simulink model "Torque_vectoring"  (R2023b)
settings: Solver=ode4  StartTime=0.0  StopTime=20  FixedStep=1e-3  RelTol=1e-3  EnableMultiTasking=on
undefined symbols (not defined in the file): A_vx, B_vx, D1, D2, LQR_DC, LQR_K, LQR_Vx_ref, N, P1, P2, par, V_ref
libraries: simulink x2, slpidlib x1
settings Model: Creator=bshyrokau  LastModifiedBy=india
settings SolverCC: AlgebraicLoopSolver=TrustRegion
settings DataIOCC: SaveOutput=off  SignalLogging=off  DSMLogging=off  SaveTime=off  ReturnWorkspaceOutputs=off
settings OptimizationCC: ReuseModelBlockBuffer=off  LifeSpan=inf
settings DebuggingCC: UnconnectedInputMsg=warning  UnconnectedOutputMsg=warning  UnconnectedLineMsg=warning  AllowSymbolicDim=off  SFUnexpectedBacktrackingDiag=warning  SFNoUnconditionalDefaultTransitionDiag=warning  SFExecutionAtInitializationDiag=none  ArithmeticOperatorsInVariantConditions=warning
settings ModelReferenceCC: EnableRefExpFcnMdlSchedulingChecks=on  PropagateSignalLabelsOutOfModel=off
settings SFSimCC: SimUseLocalCustomCode=off  CustomCodeUndefinedFunction=UseInterfaceOnly
settings RTWCC: RTWUseLocalCustomCode=off  DLArmComputeVersion=19.05
settings CodeAppCC: StateflowObjectComments=on
settings GRTTargetCC: TargetLangStandard=C89/C90 (ANSI)
settings ConfigComp: CovMetricSettings=dw  CovSaveCumulativeToWorkspaceVar=on  CovSaveSingleToWorkspaceVar=on  CovExternalEMLEnable=off
settings SimscapeCC: SimscapeNormalizeSystem=off
settings ConfigurationSet: Description=SimMechanics 2G

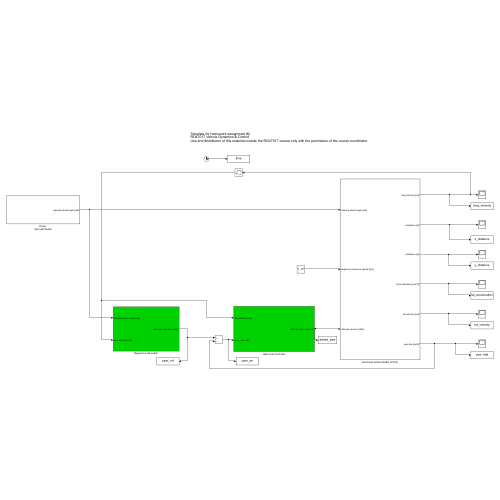
[thumbnail: Simulink's stored preview of the top-level diagram]
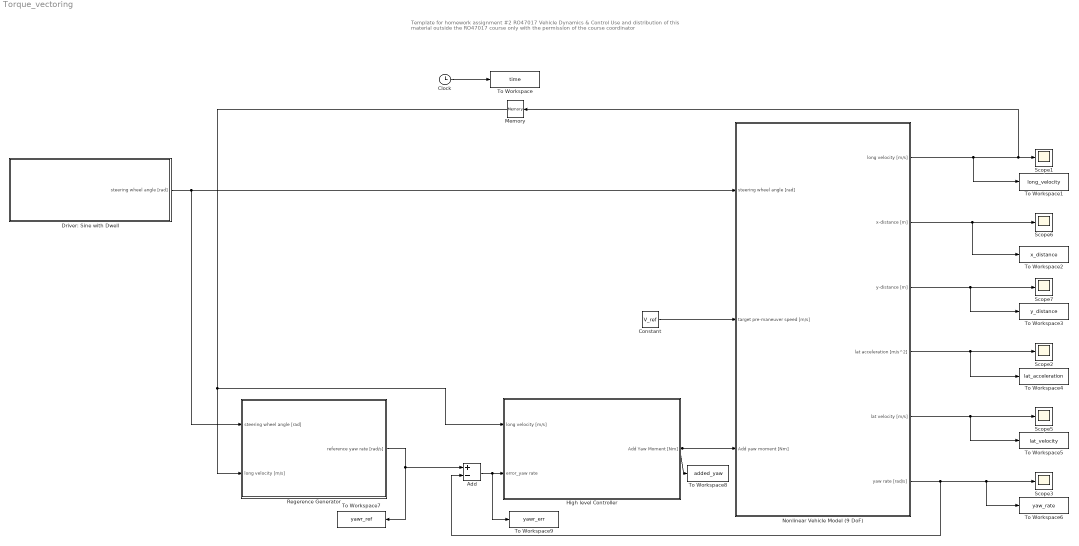
== system Torque_vectoring ==
  note: Template for homework assignment #2
      | RO47017 Vehicle Dynamics & Control
      | Use and distribution of this material outside the RO47017 course only with the permission of the course coordinator
  Add : Sum  Inputs=+-
  Clock : Clock
  Constant : Constant  Value=V_ref
  Driver: Sine with Dwell : Subsystem
  High level Controller : Subsystem
  Memory : Memory
  Nonlinear Vehicle Model (9 DoF) : Subsystem
      mask help: Simulink:masks:GenSFuncDesc_MD
      mask Help: eval('feval(''rtwprivate'',''rtwhelpview'',''rtw_sfcn_block'')');
  Regerence Generator : Subsystem
  Scope{1..3,5..7} (6 alike) : Scope
  To Workspace : ToWorkspace  VariableName=time  SampleTime=-1
  To Workspace1 : ToWorkspace  VariableName=long_velocity  SampleTime=-1
  To Workspace2 : ToWorkspace  VariableName=x_distance  SampleTime=-1
  To Workspace3 : ToWorkspace  VariableName=y_distance  SampleTime=-1
  To Workspace4 : ToWorkspace  VariableName=lat_acceleration  SampleTime=-1
  To Workspace5 : ToWorkspace  VariableName=lat_velocity  SampleTime=-1
  To Workspace6 : ToWorkspace  VariableName=yaw_rate  SampleTime=-1
  To Workspace7 : ToWorkspace  VariableName=yawr_ref  SampleTime=-1
  To Workspace8 : ToWorkspace  VariableName=added_yaw  SampleTime=-1
  To Workspace9 : ToWorkspace  VariableName=yawr_err  SampleTime=-1
  wires:
  Driver: Sine with Dwell/1(steering wheel angle [rad]) -> Regerence Generator/1(steering wheel angle [rad]), Nonlinear Vehicle Model (9 DoF)/1(steering wheel angle [rad])
  Regerence Generator/1(reference yaw rate [rad/s]) -> To Workspace7/1, Add/1
  Nonlinear Vehicle Model (9 DoF)/6(yaw rate [rad/s]) -> Add/2, Scope3/1, To Workspace6/1
  Nonlinear Vehicle Model (9 DoF)/5(lat velocity [m/s]) -> To Workspace5/1, Scope5/1
  Nonlinear Vehicle Model (9 DoF)/1(long velocity [m/s]) -> To Workspace1/1, Memory/1, Scope1/1
  Nonlinear Vehicle Model (9 DoF)/4(lat acceleration [m/s^2]) -> To Workspace4/1, Scope2/1
  Nonlinear Vehicle Model (9 DoF)/2(x-distance [m]) -> To Workspace2/1, Scope6/1
  Nonlinear Vehicle Model (9 DoF)/3(y-distance [m]) -> To Workspace3/1, Scope7/1
  Constant/1 -> Nonlinear Vehicle Model (9 DoF)/2(target pre-maneuver speed [m/s])
  Clock/1 -> To Workspace/1
  Memory/1 -> High level Controller/1(long velocity [m/s]), Regerence Generator/2(long velocity [m/s])
  Add/1 -> To Workspace9/1, High level Controller/2(error_yaw rate)
  High level Controller/1(Add Yaw Moment [Nm]) -> To Workspace8/1, Nonlinear Vehicle Model (9 DoF)/3(Add yaw moment [Nm])

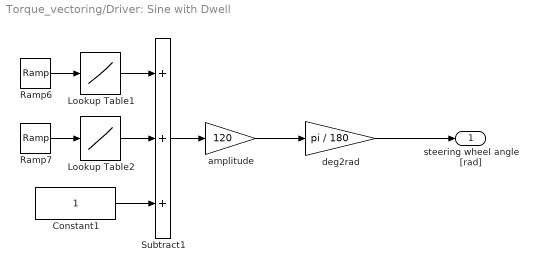
== system Torque_vectoring/Driver: Sine with Dwell ==
  Constant1 : Constant
  Lookup Table1 : Lookup  InputValues=[0:0.1:3*pi/2 3*pi/2+eps]*0.7  Table=sin([0:0.1:3*pi/2 3*pi/2+eps])  LookUpMeth=Interpolation-Use End Values  SaturateOnIntegerOverflow=off
  Lookup Table2 : Lookup  InputValues=[3*pi/2:0.1:2*pi 2*pi+eps]*0.7  Table=sin([3*pi/2:0.1:2*pi 2*pi+eps])  LookUpMeth=Interpolation-Use End Values  SaturateOnIntegerOverflow=off
  Ramp6 : simulink/Sources/Ramp  slope=pi  start=10  InitialOutput=0
  Ramp7 : simulink/Sources/Ramp  slope=pi  start=10+0.5  InitialOutput=0
  Subtract1 : Sum  Inputs=+++
  amplitude : Gain  Gain=120
  deg2rad : Gain  Gain=pi / 180
  steering wheel angle [rad] : Outport  VectorParamsAs1DForOutWhenUnconnected=off
  wires:
  Ramp6/1 -> Lookup Table1/1
  Ramp7/1 -> Lookup Table2/1
  Lookup Table2/1 -> Subtract1/2
  Lookup Table1/1 -> Subtract1/1
  Constant1/1 -> Subtract1/3
  Subtract1/1 -> amplitude/1
  amplitude/1 -> deg2rad/1
  deg2rad/1 -> steering wheel angle [rad]/1

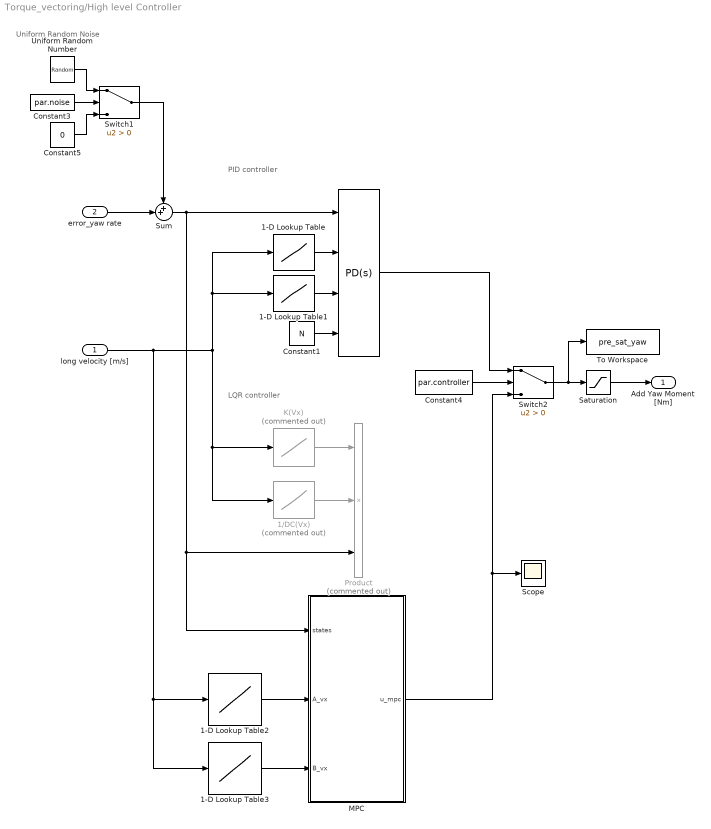
== system Torque_vectoring/High level Controller ==
  note: LQR controller
  note: Uniform Random Noise
  note: PID controller
  long velocity [m/s] : Inport
  error_yaw rate : Inport  Port=2
  " " : slpidlib/PID Controller  Controller=PD  Form=Parallel  TimeDomain=Continuous-time  UseExternalTs=off  SampleTime=-1  IntegratorMethod=Forward Euler  FilterMethod=Forward Euler  ControllerParametersSource=external  P=1  I=1  UseKiTs=off  D=0  N=100  UseFilter=on  TunerSelectOption=Transfer Function Based (PID Tuner App)  InitialConditionSource=internal  InitialConditionForIntegrator=0  InitialConditionForFilter=0  DifferentiatorICPrevScaledInput=0  ExternalReset=none  TrackingMode=off  Kt=1  LimitOutput=off  SatLimitsSource=internal  UpperSaturationLimit=inf  LowerSaturationLimit=-inf  LinearizeAsGain=on  AntiWindupMode=none  Kb=1  LimitIntegrator=off  UpperIntegratorSaturationLimit=inf  LowerIntegratorSaturationLimit=-inf  POutMin=[]  POutMax=[]  IOutMin=[]  IOutMax=[]  DOutMin=[]  DOutMax=[]  NOutMin=[]  NOutMax=[]  SumOutMin=[]  SumOutMax=[]  SaturationOutMin=[]  SaturationOutMax=[]  PParamMin=[]  PParamMax=[]  IParamMin=[]  IParamMax=[]  DParamMin=[]  DParamMax=[]  NParamMin=[]  NParamMax=[]  KbParamMin=[]  KbParamMax=[]  KtParamMin=[]  KtParamMax=[]  KbOutMin=[]  KbOutMax=[]  KtOutMin=[]  KtOutMax=[]  IntegratorOutMin=[]  IntegratorOutMax=[]  FilterOutMin=[]  FilterOutMax=[]  SumI1OutMin=[]  SumI1OutMax=[]  SumI2OutMin=[]  SumI2OutMax=[]  SumI3OutMin=[]  SumI3OutMax=[]  SumI4OutMin=[]  SumI4OutMax=[]  SumDOutMin=[]  SumDOutMax=[]  DifferentiatorOutMin=[]  DifferentiatorOutMax=[]  FilterDiffOutCoefMin=[]  FilterDiffOutCoefMax=[]  ReciprocalOutMin=[]  ReciprocalOutMax=[]  SumDenOutMin=[]  SumDenOutMax=[]  SumNumOutMin=[]  SumNumOutMax=[]  DivideOutMin=[]  DivideOutMax=[]  UdiffTsProdOutMin=[]  UdiffTsProdOutMax=[]  NTsProdOutMin=[]  NTsProdOutMax=[]  UintegralTsProdOutMin=[]  UintegralTsProdOutMax=[]  UngainTsProdOutMin=[]  UngainTsProdOutMax=[]  ClampingZeroOutDataTypeStr=Inherit: Inherit via back propagation  ClampingZeroOutMin=[]  ClampingZeroOutMax=[]  FilterDenConstantOutDataTypeStr=Inherit: Inherit via back propagation  FilterDenConstantOutMin=[]  FilterDenConstantOutMax=[]  PCopyOutDataTypeStr=Inherit: Inherit via back propagation  PCopyOutMin=[]  PCopyOutMax=[]  NCopyOutDataTypeStr=Inherit: Inherit via back propagation  NCopyOutMin=[]  NCopyOutMax=[]  IntegratorContinuousStateAttributes=''  IntegratorStateMustResolveToSignalObject=off  IntegratorRTWStateStorageClass=Auto  FilterContinuousStateAttributes=''  FilterStateMustResolveToSignalObject=off  FilterRTWStateStorageClass=Auto  ParallelPVariant=ExternalParameters  IdealPVariant=Disabled  IVariant=Disabled  DVariant=ExternalParameters  IntegratorVariant=Disabled  SatVariant=Disabled  AWVariant=Disabled  PCopyVariant=Disabled  TRVariant=Disabled  FdbkBlocksVariant=Forward  IdealPFdbkVariant=Disabled  SatFdbkVariant=Disabled  DerivativeFilterVariant=ContFilter  NVariant=ExternalParameters  NCopyVariant=Disabled  FilterICVariant=InternalICsFilter  IntegratorICVariant=Disabled  ExternalResetVariant=Disabled  TRSumVariant=Passthrough  SumFdbkVariant=Disabled  SumVariant=Sum_PD  TsampFilterVariant=InternalTs  TsampNgainVariant=Passthrough  TsampIntegralVariant=Disabled_SignalSpec  ExternalSaturationOutDataTypeStr=Inherit: Same as second input
      settings: LibrarySourceBlock=cstblocks/Linear Parameter Varying/Varying PID Controller
  1-D Lookup Table : Lookup_n-D  NumberOfTableDimensions=1  BreakpointsForDimension1=[60/3.6 100/3.6]  Table=[P1; P2]  InternalRulePriority=Speed  RndMeth=Simplest
  1-D Lookup Table1 : Lookup_n-D  NumberOfTableDimensions=1  BreakpointsForDimension1=[60/3.6 100/3.6]  Table=[D1 D2]  InternalRulePriority=Speed  RndMeth=Simplest
  1-D Lookup Table2 : Lookup_n-D  NumberOfTableDimensions=1  BreakpointsForDimension1=LQR_Vx_ref  Table=A_vx  InternalRulePriority=Speed  RndMeth=Simplest
  1-D Lookup Table3 : Lookup_n-D  NumberOfTableDimensions=1  BreakpointsForDimension1=LQR_Vx_ref  Table=B_vx  InternalRulePriority=Speed  RndMeth=Simplest
  1/DC(Vx) : Lookup_n-D  Commented=on  NumberOfTableDimensions=1  BreakpointsForDimension1=[LQR_Vx_ref]  Table=[LQR_DC]  InternalRulePriority=Speed  RndMeth=Simplest
  Constant1 : Constant  Value=N
  Constant3 : Constant  Value=par.noise
  Constant4 : Constant  Value=par.controller
  Constant5 : Constant  Value=0
  K(Vx) : Lookup_n-D  Commented=on  NumberOfTableDimensions=1  BreakpointsForDimension1=[LQR_Vx_ref]  Table=[LQR_K]  InternalRulePriority=Speed  RndMeth=Simplest
  MPC : MATLAB Function  TreatAsAtomicUnit=on
  Product : Product  Commented=on  Inputs=3
  Saturation : Saturate  UpperLimit=10000  LowerLimit=-10000
  Scope : Scope
  Sum : Sum  Inputs=++|
  Switch1 : Switch  Criteria=u2 > Threshold  SaturateOnIntegerOverflow=off  InputSameDT=off
  Switch2 : Switch  Criteria=u2 > Threshold  SaturateOnIntegerOverflow=off  InputSameDT=off
  To Workspace : ToWorkspace  VariableName=pre_sat_yaw  SampleTime=-1
  Uniform Random Number : UniformRandomNumber  Minimum=-0.0174532925  Maximum=0.0174532925  SampleTime=0
  Add Yaw Moment [Nm] : Outport  VectorParamsAs1DForOutWhenUnconnected=off
  wires:
  " "/1 -> Switch2/1
  1-D Lookup Table/1 -> " "/2
  1-D Lookup Table1/1 -> " "/3
  Constant1/1 -> " "/4
  long velocity [m/s]/1 -> 1-D Lookup Table3/1, 1-D Lookup Table2/1, 1-D Lookup Table1/1, 1-D Lookup Table/1, 1/DC(Vx)/1, K(Vx)/1
  Constant4/1 -> Switch2/2
  Saturation/1 -> Add Yaw Moment [Nm]/1
  Switch2/1 -> To Workspace/1, Saturation/1
  Uniform Random Number/1 -> Switch1/1
  Constant5/1 -> Switch1/3
  Constant3/1 -> Switch1/2
  1/DC(Vx)/1 -> Product/2
  Sum/1 -> MPC/1(states), Product/3, " "/1
  error_yaw rate/1 -> Sum/2
  Switch1/1 -> Sum/1
  K(Vx)/1 -> Product/1
  MPC/1(u_mpc) -> Scope/1, Switch2/3
  1-D Lookup Table2/1 -> MPC/2(A_vx)
  1-D Lookup Table3/1 -> MPC/3(B_vx)

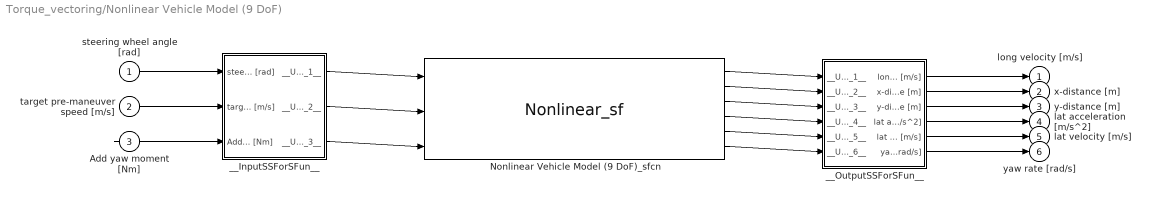
== system Torque_vectoring/Nonlinear Vehicle Model (9 DoF) ==
  steering wheel angle [rad] : Inport
  target pre-maneuver speed [m/s] : Inport  Port=2
  Add yaw moment [Nm] : Inport  Port=3
  Nonlinear Vehicle Model (9 DoF)_sfcn : S-Function  FunctionName=Nonlinear_sf  SFunctionModules=""  SFunctionDeploymentMode=off  EnableBusSupport=off  mask{rtw_sf_name=Nonlinear_sf, showVar=off}
      mask prompts: rtw_sf_name "Simulink:masks:GenSFuncName_MP"; showVar "Simulink:masks:GenSFuncShowModuleList_MP"
      mask help: Simulink:masks:GenSFuncDesc_MD
      mask init:
      | displist = '';
      | if ~strcmp(get_param(gcb, 'FunctionName'), rtw_sf_name);
      |   set_param(gcb, 'FunctionName', rtw_sf_name);
      | end
      | % Check if we are generating code
      | rtw_mode = false;
      | if strcmpi(get_param(bdroot(gcb),'SimulationStatus'),'Initializing')
      | 	rtw_mode = strcmpi(get_param(bdroot(gcb),'BuildingRTWCode'),'on') && ...
      | 		~strcmpi(get_param(bdroot(gcb),'TargetStyle'),'SimulationTarget');
      | end
      | if showVar || rtw_mode
      | 	if exist('rtwsfunc') == 2 | exist('rtwsfunc') == 6
      | 		tmplist = rtwsfunc(rtw_sf_name,gcb);
      | 		tmplist = DAStudio.message('Simulink:masks:GenSFuncListOfModules_IC', tmplist);
      | 	elseif showVar
      | 		tmplist1 = DAStudio.message('Simulink:masks:GenSFuncListOfModules_IC', '');
      |         tmplist2 = DAStudio.message('Simulink:masks:GenSFuncNotLicensed_IC');
      |         tmplist = [tmplist1 tmplist2];
      |  	end
      | end
      | if showVar
      |   displist = tmplist;
      | end
      settings: CopyFcn=|
      | if ~strcmp(get_param(gcb,'Linkstatus'),'none') && ...
      | ~strcmp(get_param(gcb,'Linkstatus'),'implicit')
      |   set_param(gcb,'LinkStatus','none');
      | end
      mask Help: eval('feval(''rtwprivate'',''rtwhelpview'',''rtw_sfcn_block'')');
      mask Display:
      | port_label('input',1,'steering wheel angle [rad]');
      | port_label('input',2,'target pre-maneuver speed [m/s]');
      | port_label('input',3,'Add yaw moment [Nm]');
      | port_label('output',1,'long velocity [m/s]');
      | port_label('output',2,'x-distance [m]');
      | port_label('output',3,'y-distance [m]');
      | port_label('output',4,'lat acceleration [m/s^2]');
      | port_label('output',5,'lat velocity [m/s]');
      | port_label('output',6,'yaw rate [rad/s]');
  __InputSSForSFun__ : Subsystem
  __OutputSSForSFun__ : Subsystem
  long velocity [m/s] : Outport  VectorParamsAs1DForOutWhenUnconnected=off
  x-distance [m] : Outport  Port=2  VectorParamsAs1DForOutWhenUnconnected=off
  y-distance [m] : Outport  Port=3  VectorParamsAs1DForOutWhenUnconnected=off
  lat acceleration [m/s^2] : Outport  Port=4  VectorParamsAs1DForOutWhenUnconnected=off
  lat velocity [m/s] : Outport  Port=5  VectorParamsAs1DForOutWhenUnconnected=off
  yaw rate [rad/s] : Outport  Port=6  VectorParamsAs1DForOutWhenUnconnected=off
  wires:
  steering wheel angle [rad]/1 -> __InputSSForSFun__/1(steering wheel angle [rad])
  target pre-maneuver speed [m/s]/1 -> __InputSSForSFun__/2(target pre-maneuver speed [m/s])
  Add yaw moment [Nm]/1 -> __InputSSForSFun__/3(Add yaw moment [Nm])
  __InputSSForSFun__/1(__UniqueOutportName__1__) -> Nonlinear Vehicle Model (9 DoF)_sfcn/1
  __InputSSForSFun__/2(__UniqueOutportName__2__) -> Nonlinear Vehicle Model (9 DoF)_sfcn/2
  __InputSSForSFun__/3(__UniqueOutportName__3__) -> Nonlinear Vehicle Model (9 DoF)_sfcn/3
  Nonlinear Vehicle Model (9 DoF)_sfcn/1 -> __OutputSSForSFun__/1(__UniqueInportName__1__)
  Nonlinear Vehicle Model (9 DoF)_sfcn/2 -> __OutputSSForSFun__/2(__UniqueInportName__2__)
  Nonlinear Vehicle Model (9 DoF)_sfcn/3 -> __OutputSSForSFun__/3(__UniqueInportName__3__)
  Nonlinear Vehicle Model (9 DoF)_sfcn/4 -> __OutputSSForSFun__/4(__UniqueInportName__4__)
  Nonlinear Vehicle Model (9 DoF)_sfcn/5 -> __OutputSSForSFun__/5(__UniqueInportName__5__)
  Nonlinear Vehicle Model (9 DoF)_sfcn/6 -> __OutputSSForSFun__/6(__UniqueInportName__6__)
  __OutputSSForSFun__/1(long velocity [m/s]) -> long velocity [m/s]/1
  __OutputSSForSFun__/2(x-distance [m]) -> x-distance [m]/1
  __OutputSSForSFun__/3(y-distance [m]) -> y-distance [m]/1
  __OutputSSForSFun__/4(lat acceleration [m/s^2]) -> lat acceleration [m/s^2]/1
  __OutputSSForSFun__/5(lat velocity [m/s]) -> lat velocity [m/s]/1
  __OutputSSForSFun__/6(yaw rate [rad/s]) -> yaw rate [rad/s]/1

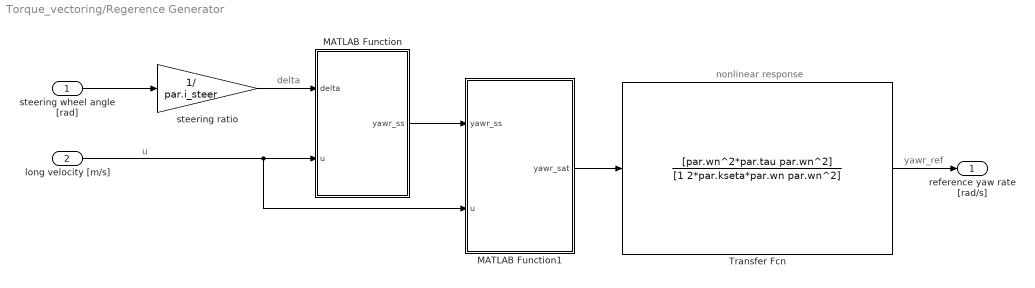
== system Torque_vectoring/Regerence Generator ==
  note: yawr_ref
  note: nonlinear response
  note: delta
  note: u
  steering wheel angle [rad] : Inport
  long velocity [m/s] : Inport  Port=2
  MATLAB Function : MATLAB Function  TreatAsAtomicUnit=on
  MATLAB Function1 : MATLAB Function  TreatAsAtomicUnit=on
  Transfer Fcn : TransferFcn  Numerator=[par.wn^2*par.tau par.wn^2]  Denominator=[1 2*par.kseta*par.wn par.wn^2]
  steering ratio : Gain  Gain=1/ par.i_steer
  reference yaw rate [rad/s] : Outport  VectorParamsAs1DForOutWhenUnconnected=off
  wires:
  steering wheel angle [rad]/1 -> steering ratio/1
  steering ratio/1 -> MATLAB Function/1(delta)
  long velocity [m/s]/1 -> MATLAB Function1/2(u), MATLAB Function/2(u)
  MATLAB Function/1(yawr_ss) -> MATLAB Function1/1(yawr_ss)
  MATLAB Function1/1(yawr_sat) -> Transfer Fcn/1
  Transfer Fcn/1 -> reference yaw rate [rad/s]/1

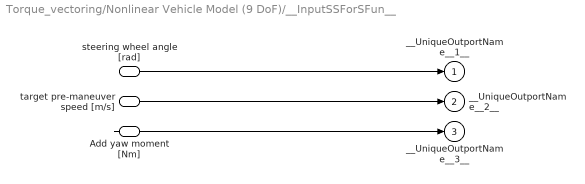
== system Torque_vectoring/Nonlinear Vehicle Model (9 DoF)/__InputSSForSFun__ ==
  steering wheel angle [rad] : Inport
  target pre-maneuver speed [m/s] : Inport  Port=2
  Add yaw moment [Nm] : Inport  Port=3
  __UniqueOutportName__1__ : Outport
  __UniqueOutportName__2__ : Outport  Port=2
  __UniqueOutportName__3__ : Outport  Port=3
  wires:
  steering wheel angle [rad]/1 -> __UniqueOutportName__1__/1
  target pre-maneuver speed [m/s]/1 -> __UniqueOutportName__2__/1
  Add yaw moment [Nm]/1 -> __UniqueOutportName__3__/1

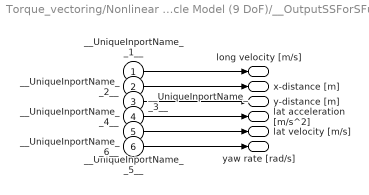
== system Torque_vectoring/Nonlinear Vehicle Model (9 DoF)/__OutputSSForSFun__ ==
  __UniqueInportName__1__ : Inport
  __UniqueInportName__2__ : Inport  Port=2
  __UniqueInportName__3__ : Inport  Port=3
  __UniqueInportName__4__ : Inport  Port=4
  __UniqueInportName__5__ : Inport  Port=5
  __UniqueInportName__6__ : Inport  Port=6
  long velocity [m/s] : Outport  VectorParamsAs1DForOutWhenUnconnected=off
  x-distance [m] : Outport  Port=2  VectorParamsAs1DForOutWhenUnconnected=off
  y-distance [m] : Outport  Port=3  VectorParamsAs1DForOutWhenUnconnected=off
  lat acceleration [m/s^2] : Outport  Port=4  VectorParamsAs1DForOutWhenUnconnected=off
  lat velocity [m/s] : Outport  Port=5  VectorParamsAs1DForOutWhenUnconnected=off
  yaw rate [rad/s] : Outport  Port=6  VectorParamsAs1DForOutWhenUnconnected=off
  wires:
  __UniqueInportName__1__/1 -> long velocity [m/s]/1
  __UniqueInportName__2__/1 -> x-distance [m]/1
  __UniqueInportName__3__/1 -> y-distance [m]/1
  __UniqueInportName__4__/1 -> lat acceleration [m/s^2]/1
  __UniqueInportName__5__/1 -> lat velocity [m/s]/1
  __UniqueInportName__6__/1 -> yaw rate [rad/s]/1

== matlab function Torque_vectoring/Regerence Generator/MATLAB Function1 ==
  data: yawr_ss input; u input; yawr_sat output; par parameter
function yawr_sat = boundary_conditions(yawr_ss,u,par)
g = par.g;
mu = par.mu;

yawr_max = 0.85*mu*g/u;

if abs(yawr_ss) > abs(yawr_max)
    yawr_sat = sign(yawr_ss)*yawr_max;
else
    yawr_sat = yawr_ss;
end

== matlab function Torque_vectoring/Regerence Generator/MATLAB Function ==
  data: delta input; u input; yawr_ss output; par parameter
function yawr_ss = bicycle_model(delta,u,par)
%Parameters
L = par.L;
g = par.g;
m = par.mass;
K = par.Kus;

%Yaw rate response
yawr_ss = u*delta/(L+K*u^2/g);

== matlab function Torque_vectoring/High level Controller/MPC ==
  data: states input; u_mpc output; par parameter; A_vx input; B_vx input
function u_mpc = fcn(states, par, A_vx, B_vx)
    A_MPC = A_Vx;
    B_MPC = B_vx;
    C_MPC = 1;
    
    % Q,R,L matrices
    Q_MPC = 1;
    R_MPC = 1;
    L_MPC = 1;
    x0 = [states; 0];

    dim.N = 15;
    dim.nx = 2;
    dim.nu = 1;
    dim.ny = 2;
    
    % Generate rate change penalty
    [A_MPC, B_MPC, C_MPC, Q_MPC, R_MPC, M_MPC, P_MPC, x0] = rate_change_pen(A_MPC, B_MPC, Q_MPC, R_MPC, L_MPC, x0);
    
    % Generate prediction matrices
    [T, S] = predmodgen(A_MPC, B_MPC, C_MPC, dim);
    
    % Generate cost function matrices
    [left, right] = costgen(T, S, Q_MPC, R_MPC, dim, x0, P_MPC, M_MPC);
    
    % Initial guess for optimization
    u0 = zeros(size(right));
    
    % Optimization options
    opts = optimoptions('quadprog', 'Display', 'off', 'Algorithm', 'active-set');
    
    % Solve quadratic program
    u_N = quadprog(left, right, [], [], [], [], [], [], u0, opts);
    
    % Output the first control action
    u_mpc = u_N(1);
end

function [A, B, C, Q, R, M, P, x0] = rate_change_pen(A, B, Q, R, L, x0)
    % Augment the state with the previous control action
    n_x = size(A, 1);
    n_u = size(B, 2);
    
    % Calculate terminal cost using the discrete algebraic Ricatti equation
    P = idare(A, B, Q, R);
    
    % Extend the system matrices
    A = [A, zeros(n_x, n_u);
         zeros(n_u, n_x), zeros(n_u, n_u)];
    B = [B; eye(n_u)];
    C = eye(n_x + n_u);
    
    % Extend the weighing matrices
    Q = [Q, zeros(n_x, n_u);
         zeros(n_u, n_x), L];
    R = R + L;
    M = -[zeros(n_x, n_u); L];
    P = [P, zeros(n_x, n_u);
         zeros(n_u, n_x), zeros(n_u, n_u)];
    
    % Extend the initial state
    x0 = [x0; zeros(n_u, 1)];
end

function [T, S] = predmodgen(A_MPC, B_MPC, C_MPC, dim)
    % Prediction matrices generation

    % Prediction matrix from initial state
    T = zeros(dim.ny * (dim.N + 1), dim.nx);
    
    for k = 0:dim.N
        Pslice = C_MPC * A_MPC^k;
        T(k * dim.ny + 1 : (k + 1) * dim.ny, :) = Pslice;
    end
    
    % Prediction matrix from input
    S = zeros(dim.ny * (dim.N + 1), dim.nu * dim.N);
    
    for k = 1:dim.N
        for i = 0:k-1
            % Calculate slice
            Sslice = C_MPC * A_MPC^(k - 1 - i) * B_MPC;
            % Update full S matrix
            S(k * dim.ny + 1 : (k + 1) * dim.ny, i * dim.nu + 1 : (i + 1) * dim.nu) = Sslice;
        end
    end
end

function [H, h] = costgen(T, S, Q, R, dim, x0, P, M)
    % Cost function generation
    
    % Define the bar matrices Qbar, Rbar, Mbar
    Qbar = blkdiag(kron(eye(dim.N), Q), P); 
    Rbar = kron(eye(dim.N), R);
    Mbar = [kron(eye(dim.N), M); zeros(dim.nx, dim.N * dim.nu)];
    
    % Calculate H and h
    H = Rbar + S' * Qbar * S + 2 * S' * Mbar;  
    h = S' * Qbar * T * x0 + Mbar' * T * x0;
end







% function u_mpc = fcn(states, T,S,Q_MPC,R_MPC,dim,P_MPC,M_MPC)
%     x0 = [states;0];
%     [left,right]=costgen(T,S,Q_MPC,R_MPC,dim,x0,P_MPC,M_MPC);
%     u0 = zeros(size(right));
% %     u_mpc = 0;
%     opts = optimoptions('quadprog','Display','off','Algorithm','active-set');
%     u_N = quadprog(left,right,[],[],[],[],[],[],u0,opts);
%     u_mpc = u_N(1);
% end
% 
% function [H,h]=costgen(T,S,Q,R,dim,x0,P,M)
%     % Cost function generation
%     % Converts a cost function of the form:
%     % V_N(x(0),u_n) = 0.5*sum_{0,N-1}(x'Qx + u'Ru + 2x'Mu) + 0.5x_N'Px_N
%     % into a form only dependent on u_N:
%     % V_N(u_N) = 0.5u'Hu + h'u + c
% 
%     if nargin == 6
%         M = zeros(dim.nx,dim.nu);
%         P = Q;
%     end
% 
%     % Define the bar matrices Qbar, Rbar, Mbar
%     Qbar = blkdiag(kron(eye(dim.N),Q),P); 
%     Rbar = kron(eye(dim.N),R);
%     Mbar = [kron(eye(dim.N),M);zeros(dim.nx,dim.N*dim.nu)];
% 
%     % Calculate H,h,c
%     H = (Rbar + S'*Qbar*S + 2*S'*Mbar);  
% 
%     % Stabilizing version
%     h = (S'*Qbar*T*x0 + Mbar'*T*x0);
% end
